simulink model "SystemModel"  (R2018a)
settings: Solver=FixedStepAuto  StartTime=0.0  StopTime=sm.T  FixedStep=sm.Ts  RelTol=1e-3
StopFcn:
  | stopCallback
undefined symbols (not defined in the file or in its folder): Controller, controller_cl, ctrl, gradientBased, GradientBasedUpdateLaw, ILCUpdate, ILCUpdateLaw, iterationPhase_enum, plant, simulationPhase_enum, smoothTransition, SmoothTransition, updateLaw_cd
libraries: simulink x3, reelInOut x1, reelOut x1, controllerComponents x1, determineIterationPhase_ul x1, determineSimulationPhase_ul x1, findClosestPointOnPath_cl x1, getTargetPoint x1, gradient_ul x1, persistentExcitation_ul x1, trustRegion_ul x1, optimumBased x1
settings Model: SimulationMode=rapid-accelerator  PauseTimes=78.131  SnapshotBufferSize=2  SnapshotInterval=1  ExtModeTrigDuration=100  Creator=M.Cobb  LastModifiedBy=mitch
settings DataIOCC: SaveFormat=StructureWithTime  SaveOutput=off  StateSaveName=tmp_raccel_xout
settings OptimizationCC: DefaultParameterBehavior=Inlined  EfficientMapNaN2IntZero=off
settings DebuggingCC: InheritedTsInSrcMsg=none  AllowedUnitSystems=SI,SI (extended)
settings HardwareCC: TargetBitPerPointer=64  TargetBitPerSizeT=64  TargetBitPerPtrDiffT=64  TargetLongLongMode=on  TargetIntDivRoundTo=Zero  TargetEndianess=LittleEndian  TargetWordSize=64  TargetHWDeviceType=MATLAB Host  ProdEqTarget=off
settings RTWCC: SystemTargetFile=raccel.tlc  TemplateMakefile=raccel_default_tmf  RTWVerbose=off  RTWUseSimCustomCode=on
settings CodeAppCC: GenerateComments=off  MaxIdLength=128  MangleLength=10  SimulinkBlockComments=off
settings RaccelTargetCC: GeneratePreprocessorConditionals=Use local settings  MultiInstanceERTCode=off  ENABLE_SLEXEC_SSBRIDGE=11  RTWCAPIParams=on

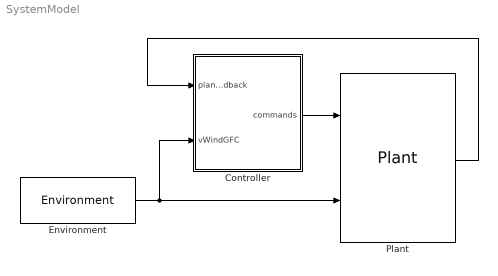
== system SystemModel ==
  Controller : Subsystem  AncestorBlock=controller_cl/Controller  Variant=on  mask{actVariant=Smooth Transition}
      mask prompts: actVariant "Select Active Variant"
      mask TypeOptions actVariant: Reel Out | Reel In & Out | Smooth Transition
      mask Callback actVariant: setControllerVariant
      mask Display:
      | text(0.5, 0.9, get(gcbh,'actVariant'), 'horizontalAlignment', 'center')
      | port_label('input',1,'feedback')
      | port_label('input',2,'environment')
      | port_label('output',1,'commands')
  Environment : environment_cl/Environment
  Plant : plant_cl/Plant
  wires:
  Environment/1 -> Controller/2(vWindGFC), Plant/2
  Controller/1(commands) -> Plant/1
  Plant/1 -> Controller/1(plantFeedback)

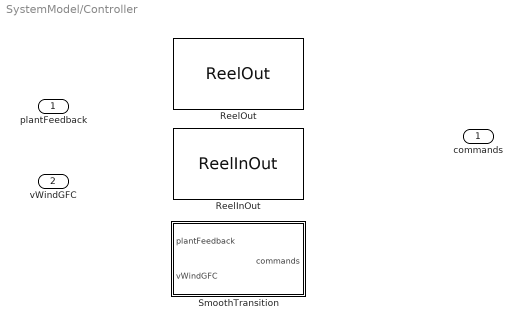
== system SystemModel/Controller ==
  plantFeedback : Inport  OutDataTypeStr=Bus: busPlantFeedback
  vWindGFC : Inport  Port=2
  ReelInOut : reelInOut/ReelInOut  VariantControl=variantReelInOut
  ReelOut : reelOut/ReelOut  VariantControl=variantReelOut
  SmoothTransition : Subsystem  AncestorBlock=smoothTransition/SmoothTransition  VariantControl=variantSmoothTransition
  commands : Outport  OutDataTypeStr=Bus: busControllerOutput

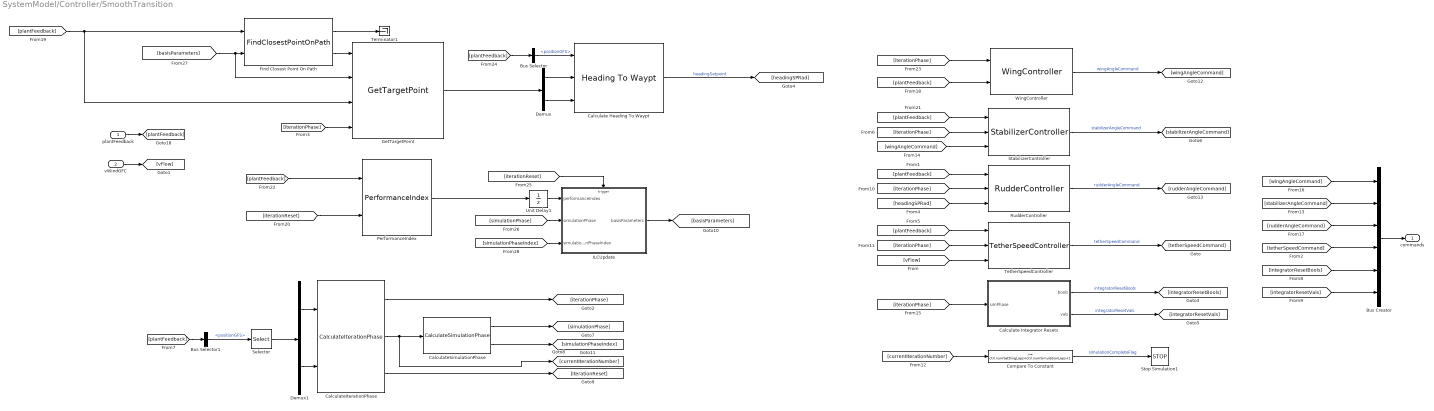
== system SystemModel/Controller/SmoothTransition ==
  plantFeedback : Inport  OutDataTypeStr=Bus: busPlantFeedback
  vWindGFC : Inport  Port=2
  Bus Creator : BusCreator  Inputs=6  OutDataTypeStr=Bus: busControllerOutput
  Bus Selector : BusSelector  OutputSignals=positionGFS
  Bus Selector1 : BusSelector  OutputSignals=positionGFS
  Calculate Heading To Waypt : controllerComponents/Heading To Waypt
  Calculate Integrator Resets : Subsystem
  CalculateIterationPhase : determineIterationPhase_ul/CalculateIterationPhase
  CalculateSimulationPhase : determineSimulationPhase_ul/CalculateSimulationPhase
  Compare To Constant : simulink/Logic and Bit Operations/Compare To Constant  relop=>=  const=ctrl.numSettlingLaps+ctrl.numSimulationLaps+1  OutDataTypeStr=boolean
  Demux : Demux  Outputs=2
  Demux1 : Demux  Outputs=2
  Find Closest Point On Path : findClosestPointOnPath_cl/FindClosestPointOnPath
  GetTargetPoint : getTargetPoint/GetTargetPoint
  ILCUpdate : Subsystem  AncestorBlock=ILCUpdate/ILCUpdate
  PerformanceIndex : PerformanceIndex/PerformanceIndex
  RudderController : rudderController/RudderController
  Selector : Selector  InputPortWidth=3  IndexOptions=Index vector (dialog)  Indices=[1 2]  OutputSizes=1
  StabilizerController : stabilizerController_ul/StabilizerController
  Stop Simulation1 : Stop
  Terminator1 : Terminator
  TetherSpeedController : tetherSpeedController/TetherSpeedController
  Unit Delay1 : UnitDelay  SampleTime=-1
  WingController : wingController/WingController
  commands : Outport  OutDataTypeStr=Bus: busControllerOutput
  wires:
  [simulationPhaseIndex] -> ILCUpdate/3(simulationPhaseIndex)
  CalculateSimulationPhase/2 -> [simulationPhaseIndex]
  ILCUpdate/1(basisParameters) -> [basisParameters]
  [simulationPhase] -> ILCUpdate/2(simulationPhase)
  [iterationReset] -> ILCUpdate/Trigger
  PerformanceIndex/1 -> Unit Delay1/1
  [plantFeedback] -> PerformanceIndex/1
  [iterationReset] -> PerformanceIndex/2
  CalculateIterationPhase/3 -> [iterationReset]
  [iterationPhase] -> GetTargetPoint/4
  GetTargetPoint/1 -> Demux/1
  CalculateIterationPhase/1 -> [iterationPhase]
  CalculateSimulationPhase/1 -> [simulationPhase]
  Selector/1 -> Demux1/1
  Demux1/2 -> CalculateIterationPhase/2
  Demux1/1 -> CalculateIterationPhase/1
  Bus Selector1/1 -> Selector/1  "<positionGFS>"
  [plantFeedback] -> Bus Selector1/1
  CalculateIterationPhase/2 -> CalculateSimulationPhase/1, [currentIterationNumber]
  Demux/2 -> Calculate Heading To Waypt/3
  Demux/1 -> Calculate Heading To Waypt/2
  Bus Selector/1 -> Calculate Heading To Waypt/1  "<positionGFS>"
  [plantFeedback] -> Bus Selector/1
  Find Closest Point On Path/1 -> Terminator1/1
  [basisParameters] -> Find Closest Point On Path/2, GetTargetPoint/2
  Find Closest Point On Path/2 -> GetTargetPoint/1
  [plantFeedback] -> Find Closest Point On Path/1, GetTargetPoint/3
  plantFeedback/1 -> [plantFeedback]
  vWindGFC/1 -> [vFlow]
  Bus Creator/1 -> commands/1
  [currentIterationNumber] -> Compare To Constant/1
  Compare To Constant/1 -> Stop Simulation1/1  "simulationCompleteFlag"
  Calculate Heading To Waypt/1 -> [headingSPRad]  "headingSetpoint"
  RudderController/1 -> [rudderAngleCommand]  "rudderAngleCommand"
  TetherSpeedController/1 -> [tetherSpeedCommand]  "tetherSpeedCommand"
  [plantFeedback] -> WingController/2
  WingController/1 -> [wingAngleCommand]  "wingAngleCommand"
  [iterationPhase] -> WingController/1
  [iterationPhase] -> Calculate Integrator Resets/1(simPhase)
  Calculate Integrator Resets/1(bools) -> [integratorResetBools]  "integratorResetBools"
  Calculate Integrator Resets/2(vals) -> [integratorResetVals]  "integratorResetVals"
  [vFlow] -> TetherSpeedController/3
  [plantFeedback] -> TetherSpeedController/1
  [iterationPhase] -> TetherSpeedController/2
  [integratorResetVals] -> Bus Creator/6
  [integratorResetBools] -> Bus Creator/5
  [tetherSpeedCommand] -> Bus Creator/4
  [rudderAngleCommand] -> Bus Creator/3
  [wingAngleCommand] -> Bus Creator/1
  StabilizerController/1 -> [stabilizerAngleCommand]  "stabilizerAngleCommand"
  [stabilizerAngleCommand] -> Bus Creator/2
  [plantFeedback] -> RudderController/1
  [headingSPRad] -> RudderController/3
  [iterationPhase] -> RudderController/2
  [iterationPhase] -> StabilizerController/2
  [plantFeedback] -> StabilizerController/1
  [wingAngleCommand] -> StabilizerController/3
  Unit Delay1/1 -> ILCUpdate/1(performanceIndex)

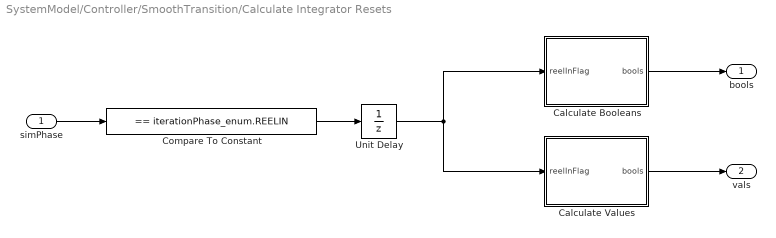
== system SystemModel/Controller/SmoothTransition/Calculate Integrator Resets ==
  simPhase : Inport
  Calculate Booleans : Subsystem
  Calculate Values : Subsystem
  Compare To Constant : simulink/Logic and Bit Operations/Compare To Constant  relop===  const=iterationPhase_enum.REELIN  OutDataTypeStr=boolean
  Unit Delay : UnitDelay  InitialCondition=false  SampleTime=-1
  bools : Outport
  vals : Outport  Port=2
  wires:
  Unit Delay/1 -> Calculate Booleans/1(reelInFlag), Calculate Values/1(reelInFlag)
  simPhase/1 -> Compare To Constant/1
  Compare To Constant/1 -> Unit Delay/1
  Calculate Booleans/1(bools) -> bools/1
  Calculate Values/1(bools) -> vals/1

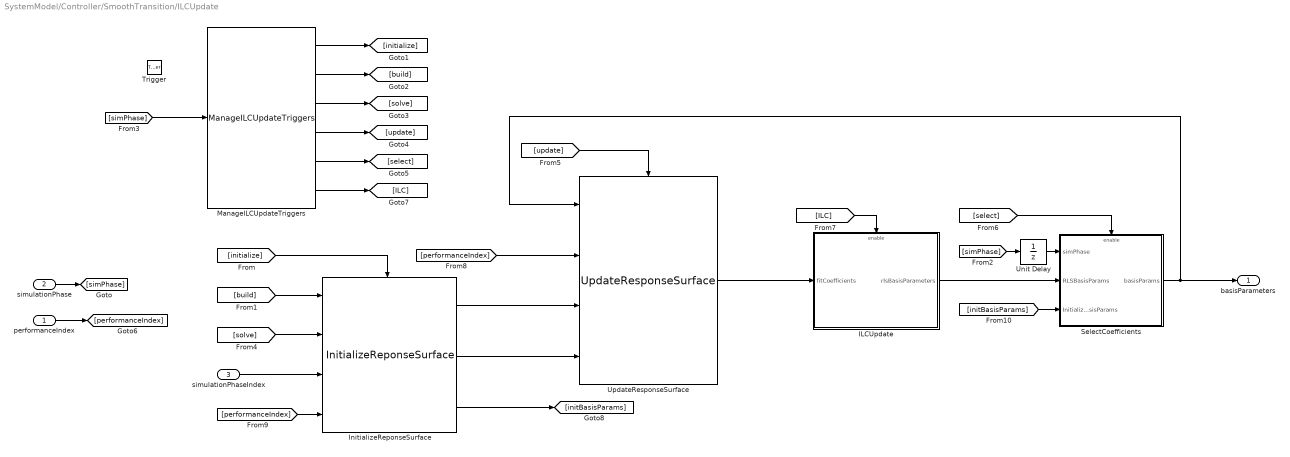
== system SystemModel/Controller/SmoothTransition/ILCUpdate ==
  performanceIndex : Inport
  simulationPhase : Inport  Port=2  OutDataTypeStr=Enum: simulationPhase_enum
  simulationPhaseIndex : Inport  Port=3
  Trigger : TriggerPort  VariantControl=Variant  InitialTriggerSignalState=positive  PortDimensions=1
  ILCUpdate : Subsystem
  InitializeReponseSurface : initializeResponseSurface_cd/InitializeReponseSurface
  ManageILCUpdateTriggers : manageILCTriggers_ul/ManageILCUpdateTriggers
  SelectCoefficients : Subsystem
  Unit Delay : UnitDelay  InitialCondition=simulationPhase_enum.SETTLING  SampleTime=-1
  UpdateResponseSurface : updateResponseSurface_ul/UpdateResponseSurface
  basisParameters : Outport  InitialOutput=[ctrl.width ctrl.height]*pi/180
  wires:
  [performanceIndex] -> UpdateResponseSurface/2
  Unit Delay/1 -> SelectCoefficients/1(simPhase)
  SelectCoefficients/1(basisParams) -> basisParameters/1, UpdateResponseSurface/1
  [initBasisParams] -> SelectCoefficients/3(InitializationBasisParams)
  InitializeReponseSurface/3 -> [initBasisParams]
  ILCUpdate/1(rlsBasisParameters) -> SelectCoefficients/2(RLSBasisParams)
  [performanceIndex] -> InitializeReponseSurface/4
  performanceIndex/1 -> [performanceIndex]
  simulationPhaseIndex/1 -> InitializeReponseSurface/3
  InitializeReponseSurface/2 -> UpdateResponseSurface/4
  InitializeReponseSurface/1 -> UpdateResponseSurface/3
  UpdateResponseSurface/1 -> ILCUpdate/1(fitCoefficients)
  simulationPhase/1 -> [simPhase]
  [simPhase] -> Unit Delay/1
  [simPhase] -> ManageILCUpdateTriggers/1
  ManageILCUpdateTriggers/1 -> [initialize]
  ManageILCUpdateTriggers/2 -> [build]
  ManageILCUpdateTriggers/6 -> [ILC]
  ManageILCUpdateTriggers/5 -> [select]
  ManageILCUpdateTriggers/4 -> [update]
  ManageILCUpdateTriggers/3 -> [solve]
  [initialize] -> InitializeReponseSurface/Enable
  [build] -> InitializeReponseSurface/1
  [solve] -> InitializeReponseSurface/2
  [update] -> UpdateResponseSurface/Enable
  [select] -> SelectCoefficients/Enable
  [ILC] -> ILCUpdate/Enable

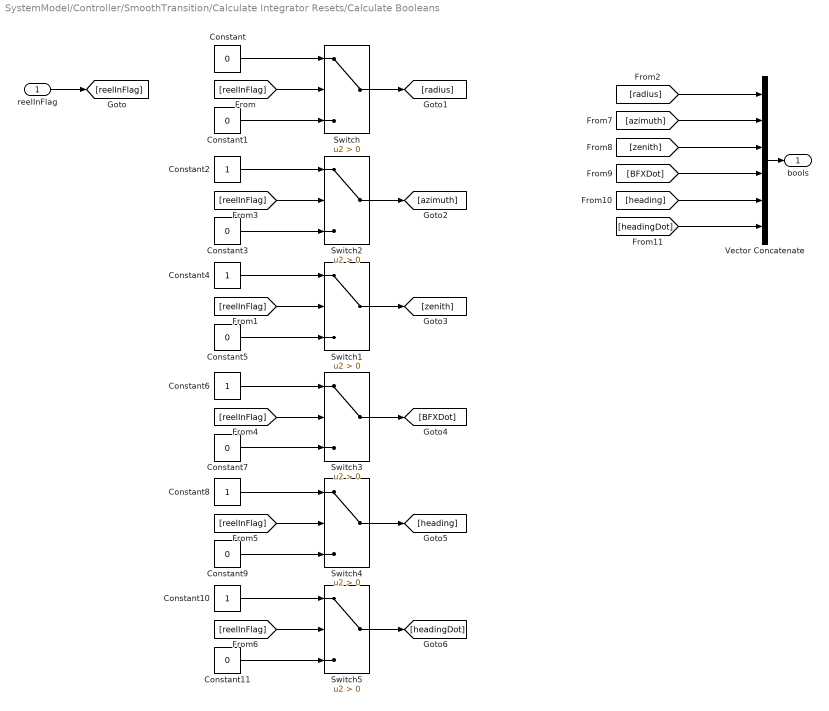
== system SystemModel/Controller/SmoothTransition/Calculate Integrator Resets/Calculate Booleans ==
  reelInFlag : Inport
  Constant{,1,3,5,7,9,11} (7 alike) : Constant  Value=0  OutDataTypeStr=boolean
  Constant{2,4,6,8,10} (5 alike) : Constant  OutDataTypeStr=boolean
  Switch{,1..5} (6 alike) : Switch  Criteria=u2 > Threshold
  Vector Concatenate : Concatenate  NumInputs=6
  bools : Outport
  wires:
  [radius] -> Vector Concatenate/1
  [headingDot] -> Vector Concatenate/6
  [heading] -> Vector Concatenate/5
  [BFXDot] -> Vector Concatenate/4
  [zenith] -> Vector Concatenate/3
  [azimuth] -> Vector Concatenate/2
  Constant8/1 -> Switch4/1
  Switch4/1 -> [heading]
  Constant9/1 -> Switch4/3
  [reelInFlag] -> Switch4/2
  Constant5/1 -> Switch1/3
  Constant4/1 -> Switch1/1
  [reelInFlag] -> Switch1/2
  [reelInFlag] -> Switch/2
  Switch1/1 -> [zenith]
  [reelInFlag] -> Switch5/2
  Switch5/1 -> [headingDot]
  Constant10/1 -> Switch5/1
  Constant11/1 -> Switch5/3
  Constant/1 -> Switch/1
  Switch/1 -> [radius]
  Constant1/1 -> Switch/3
  Constant7/1 -> Switch3/3
  [reelInFlag] -> Switch3/2
  Constant6/1 -> Switch3/1
  Switch3/1 -> [BFXDot]
  Vector Concatenate/1 -> bools/1
  Constant2/1 -> Switch2/1
  Constant3/1 -> Switch2/3
  Switch2/1 -> [azimuth]
  [reelInFlag] -> Switch2/2
  reelInFlag/1 -> [reelInFlag]

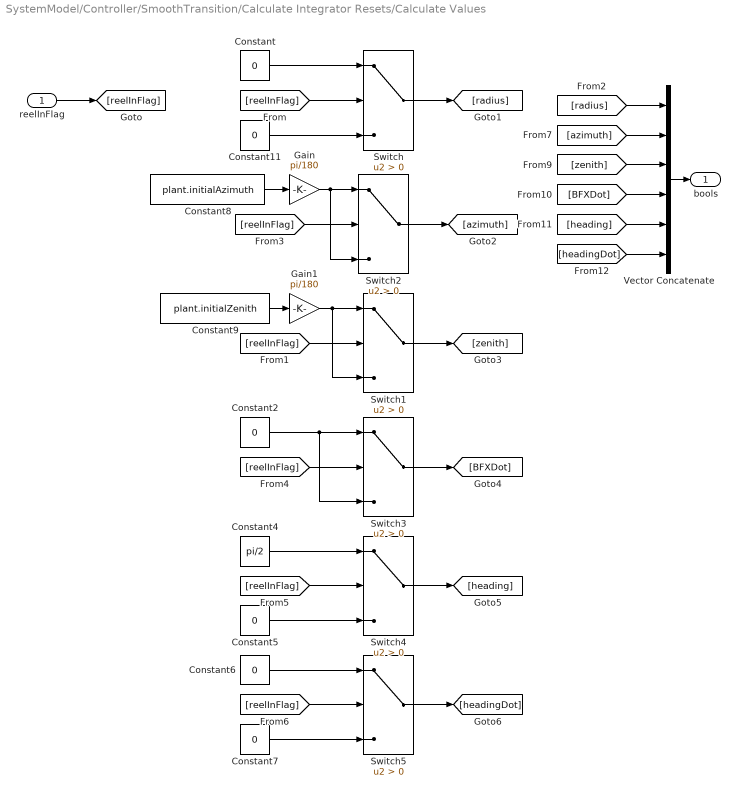
== system SystemModel/Controller/SmoothTransition/Calculate Integrator Resets/Calculate Values ==
  reelInFlag : Inport
  Constant{,2,5..7,11} (6 alike) : Constant  Value=0  OutDataTypeStr=double
  Constant4 : Constant  Value=pi/2  OutDataTypeStr=double
  Constant8 : Constant  Value=plant.initialAzimuth  OutDataTypeStr=double
  Constant9 : Constant  Value=plant.initialZenith  OutDataTypeStr=double
  Gain : Gain  Gain=pi/180
  Gain1 : Gain  Gain=pi/180
  Switch{,1..5} (6 alike) : Switch  Criteria=u2 > Threshold
  Vector Concatenate : Concatenate  NumInputs=6
  bools : Outport
  wires:
  Constant4/1 -> Switch4/1
  Switch4/1 -> [heading]
  Constant5/1 -> Switch4/3
  [reelInFlag] -> Switch4/2
  Gain1/1 -> Switch1/3, Switch1/1
  Constant9/1 -> Gain1/1
  [reelInFlag] -> Switch1/2
  [reelInFlag] -> Switch/2
  Switch1/1 -> [zenith]
  [radius] -> Vector Concatenate/1
  [reelInFlag] -> Switch5/2
  Switch5/1 -> [headingDot]
  Constant6/1 -> Switch5/1
  Constant7/1 -> Switch5/3
  Constant/1 -> Switch/1
  [BFXDot] -> Vector Concatenate/4
  Switch/1 -> [radius]
  Constant11/1 -> Switch/3
  Constant2/1 -> Switch3/3, Switch3/1
  [reelInFlag] -> Switch3/2
  Switch3/1 -> [BFXDot]
  Vector Concatenate/1 -> bools/1
  [azimuth] -> Vector Concatenate/2
  [zenith] -> Vector Concatenate/3
  [heading] -> Vector Concatenate/5
  Constant8/1 -> Gain/1
  Gain/1 -> Switch2/3, Switch2/1
  Switch2/1 -> [azimuth]
  [reelInFlag] -> Switch2/2
  [headingDot] -> Vector Concatenate/6
  reelInFlag/1 -> [reelInFlag]

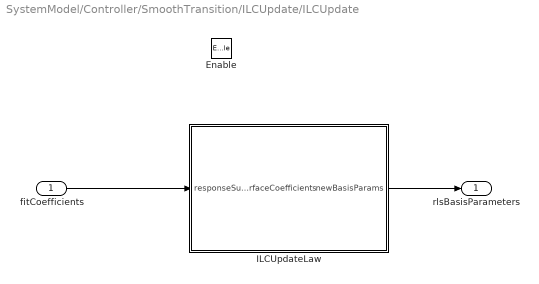
== system SystemModel/Controller/SmoothTransition/ILCUpdate/ILCUpdate ==
  fitCoefficients : Inport
  Enable : EnablePort
  ILCUpdateLaw : Subsystem  AncestorBlock=updateLaw_cd/ILCUpdateLaw  Variant=on
  rlsBasisParameters : Outport
  wires:
  ILCUpdateLaw/1(newBasisParams) -> rlsBasisParameters/1
  fitCoefficients/1 -> ILCUpdateLaw/1(responseSurfaceCoefficients)

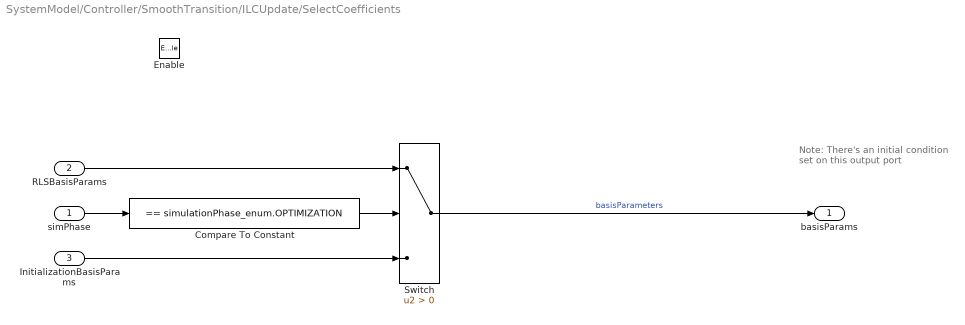
== system SystemModel/Controller/SmoothTransition/ILCUpdate/SelectCoefficients ==
  note: Note: There's an initial condition
      | set on this output port
  simPhase : Inport
  RLSBasisParams : Inport  Port=2
  InitializationBasisParams : Inport  Port=3
  Enable : EnablePort
  Compare To Constant : simulink/Logic and Bit Operations/Compare To Constant  relop===  const=simulationPhase_enum.OPTIMIZATION  OutDataTypeStr=boolean
  Switch : Switch  Criteria=u2 > Threshold
  basisParams : Outport  InitialOutput=[ctrl.width ctrl.height]*pi/180
  wires:
  Compare To Constant/1 -> Switch/2
  RLSBasisParams/1 -> Switch/1
  InitializationBasisParams/1 -> Switch/3
  simPhase/1 -> Compare To Constant/1
  Switch/1 -> basisParams/1  "basisParameters"

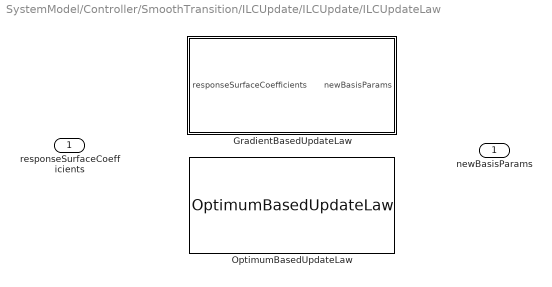
== system SystemModel/Controller/SmoothTransition/ILCUpdate/ILCUpdate/ILCUpdateLaw ==
  responseSurfaceCoefficients : Inport
  GradientBasedUpdateLaw : Subsystem  AncestorBlock=gradientBased/GradientBasedUpdateLaw  VariantControl=variantGradientBased
  OptimumBasedUpdateLaw : optimumBased/OptimumBasedUpdateLaw  VariantControl=variantOptimumBased
  newBasisParams : Outport

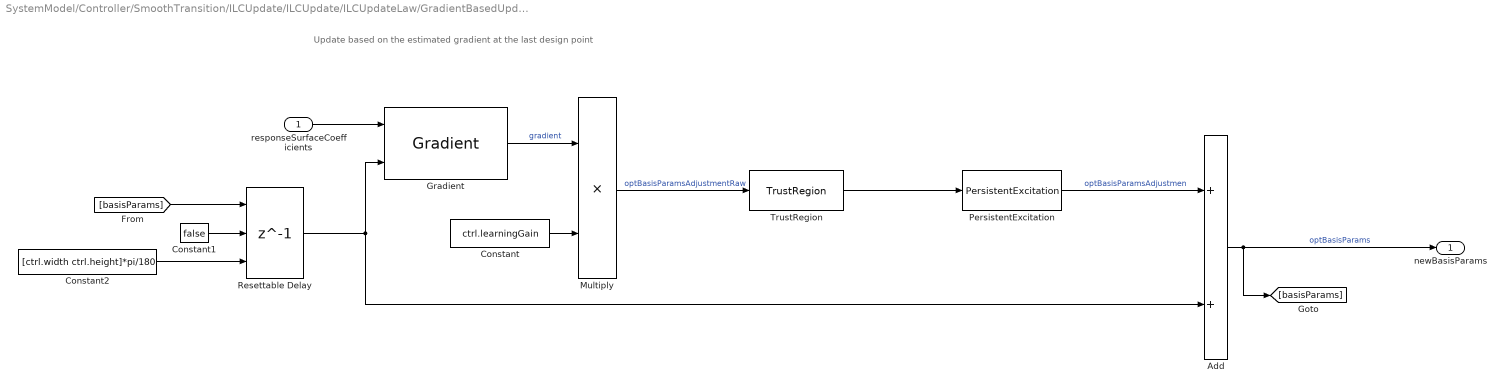
== system SystemModel/Controller/SmoothTransition/ILCUpdate/ILCUpdate/ILCUpdateLaw/GradientBasedUpdateLaw ==
  note: Update based on the estimated gradient at the last design point
  responseSurfaceCoefficients : Inport
  Add : Sum
  Constant : Constant  Value=ctrl.learningGain
  Constant1 : Constant  Value=false
  Constant2 : Constant  Value=[ctrl.width ctrl.height]*pi/180
  Gradient : gradient_ul/Gradient
  Multiply : Product
  PersistentExcitation : persistentExcitation_ul/PersistentExcitation
  Resettable Delay : Delay  DelayLength=1  InitialConditionSource=Input port  ExternalReset=Rising
      settings: InputPortMap=u0,r5,p4
  TrustRegion : trustRegion_ul/TrustRegion
  newBasisParams : Outport
  wires:
  PersistentExcitation/1 -> Add/1  "optBasisParamsAdjustmen"
  Constant2/1 -> Resettable Delay/3
  Constant1/1 -> Resettable Delay/2
  [basisParams] -> Resettable Delay/1
  Add/1 -> newBasisParams/1, [basisParams]  "optBasisParams"
  TrustRegion/1 -> PersistentExcitation/1
  Constant/1 -> Multiply/2
  Gradient/1 -> Multiply/1  "gradient"
  Multiply/1 -> TrustRegion/1  "optBasisParamsAdjustmentRaw"
  Resettable Delay/1 -> Gradient/2, Add/2
  responseSurfaceCoefficients/1 -> Gradient/1
